simulink model "indivresea"  (R2023a)
settings: Solver=VariableStepAuto  StartTime=0.0  StopTime=10  RelTol=1e-3
libraries: simulink x2, commchan3 x1, simulink_extras x1
settings Model: Creator=kimyounghwan  LastModifiedBy=BRAIN

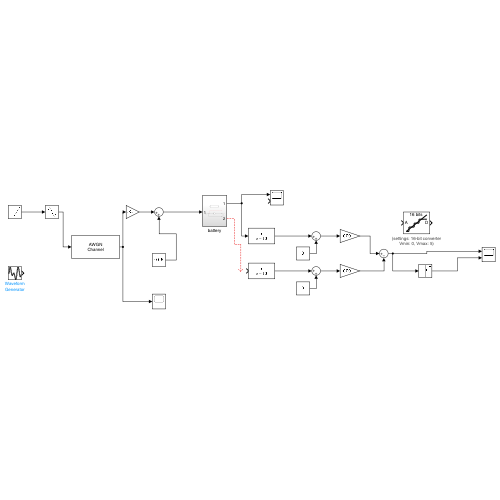
[thumbnail: Simulink's stored preview of the top-level diagram]
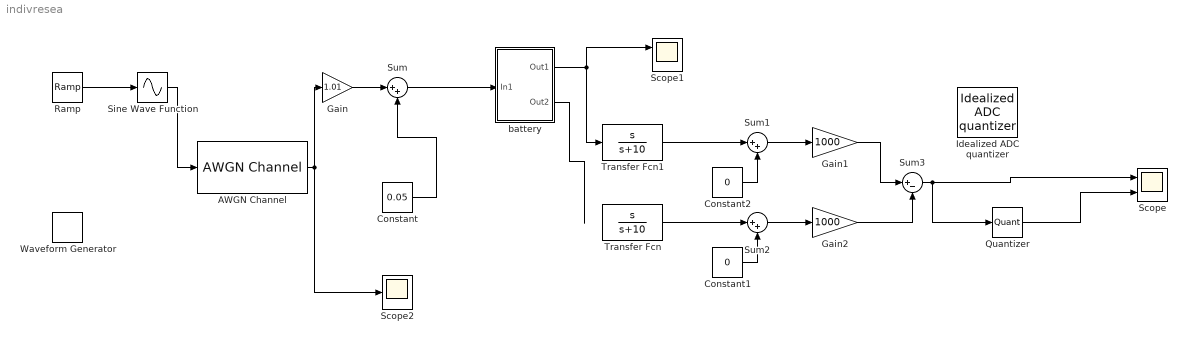
== system indivresea ==
  AWGN Channel : commchan3/AWGN Channel  LegacyMode=off  NoiseMethod="Signal to noise ratio  (SNR)"  noiseMode="Signal to noise ratio  (SNR)"  EbNo=10  EsNo=10  SNR=30  BitsPerSymbol=1  SignalPower=0.1  SamplesPerSymbol=1  SymbolPeriod=1  VarianceSource=Parameter  Variance=1  RandomStream=Global stream  Seed=67  SimulateUsing=Code generation
  Constant : Constant  Value=0.05
  Constant1 : Constant  Value=0
  Constant2 : Constant  Value=0
  Gain : Gain  Gain=1.01
  Gain1 : Gain  Gain=1000
  Gain2 : Gain  Gain=1000
  Idealized ADC quantizer : simulink_extras/Additional Discrete/Idealized ADC quantizer  NumberOfConverterBits=16  Vmin=0  Vmax=5  OutputDataType=int16  OutputNegativeValues=on
  Quantizer : Quantizer  QuantizationInterval=0.05
  Ramp : simulink/Sources/Ramp  slope=1  start=0  InitialOutput=0
  Scope : Scope  NumInputPorts=2
  Scope1 : Scope  NumInputPorts=2
  Scope2 : Scope
  Sine Wave Function : Sin  TimeSource=Use external signal  SampleTime=0
  Sum : Sum  Inputs=|++
  Sum1 : Sum  Inputs=|++
  Sum2 : Sum  Inputs=|++
  Sum3 : Sum  Inputs=|+-
  Transfer Fcn : TransferFcn  Numerator=[1 0]  Denominator=[1 10]
  Transfer Fcn1 : TransferFcn  Numerator=[1 0]  Denominator=[1 10]
  Waveform Generator : simulink/Sources/Waveform Generator  OutMin=[]  OutMax=[]  OutDataTypeStr=double  SelectedSignal=1  Signals=sin(1,0.5,0)  BlockNames=MultiportSwitch_743969d7ea52468  SampleTime=0.1
  battery : Subsystem
  wires:
  Gain/1 -> Sum/1
  Sum/1 -> battery/1(In1)
  battery/2(Out2) -> ?
  battery/1(Out1) -> Transfer Fcn1/1, Scope1/1
  Constant/1 -> Sum/2
  Sum1/1 -> Gain1/1
  Sum2/1 -> Gain2/1
  Constant2/1 -> Sum1/2
  Constant1/1 -> Sum2/2
  Gain2/1 -> Sum3/2
  Gain1/1 -> Sum3/1
  Sum3/1 -> Quantizer/1, Scope/1
  Transfer Fcn1/1 -> Sum1/1
  Transfer Fcn/1 -> Sum2/1
  Quantizer/1 -> Scope/2
  Ramp/1 -> Sine Wave Function/1
  Sine Wave Function/1 -> AWGN Channel/1
  AWGN Channel/1 -> Scope2/1, Gain/1

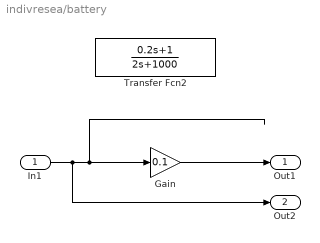
== system indivresea/battery ==
  In1 : Inport
  Gain : Gain  Gain=0.1
  Transfer Fcn2 : TransferFcn  Numerator=[0.2 1]  Denominator=[2 1000]
  Out1 : Outport
  Out2 : Outport  Port=2
  wires:
  In1/1 -> Out2/1, Gain/1
  Gain/1 -> Out1/1
